simulink model "adas"  (R2022a)
settings: Solver=ode3  StartTime=0.0  StopTime=100  FixedStep=0.02  RelTol=1e-3  EnableMultiTasking=on
undefined symbols (not defined in the file): kd, kp
libraries: simulink x1
settings Model: ExtModeTrigDuration=2  Creator=hp  LastModifiedBy=hp
settings DataIOCC: TimeSaveName=HIL  OutputSaveName=HIL  SignalLoggingName=HILout  DSMLoggingName=HILout
settings OptimizationCC: EnhancedBackFolding=on  PassReuseOutputArgsAs=Individual arguments  ZeroExternalMemoryAtStartup=off  ZeroInternalMemoryAtStartup=off  MaxStackSize=64  OptimizeBlockOrder=speed  DifferentSizesBufferReuse=on  OptimizationCustomize=off  EfficientTunableParamExpr=on
settings DebuggingCC: ParameterTunabilityLossMsg=error
settings HardwareCC: ProdBitPerInt=16  ProdBitPerPointer=16  ProdBitPerSizeT=16  ProdBitPerPtrDiffT=16  ProdLargestAtomicFloat=None  ProdWordSize=8  ProdHWDeviceType=Atmel->AVR
settings SFSimCC: MATLABDynamicMemAlloc=off
settings RTWCC: SystemTargetFile=ert.tlc  HardwareBoard=Arduino Uno  TemplateMakefile=ert_default_tmf  Toolchain=Arduino AVR  BuildConfiguration=Faster Runs  PortableWordSizes=on
settings CodeAppCC: ForceParamTrailComments=on  IgnoreCustomStorageClasses=off  OperatorAnnotations=on  SimulinkDataObjDesc=on  SFDataObjDesc=on  InsertBlockDesc=on
settings ERTTargetCC: SupportContinuousTime=on  SupportVariableSizeSignals=on  ExtModeTransport=3  ExtModeStaticAlloc=on  ExtModeStaticAllocSize=250  ExtModeMexFile=ext_xcp  ExtModeIntrfLevel=Level2 - Open

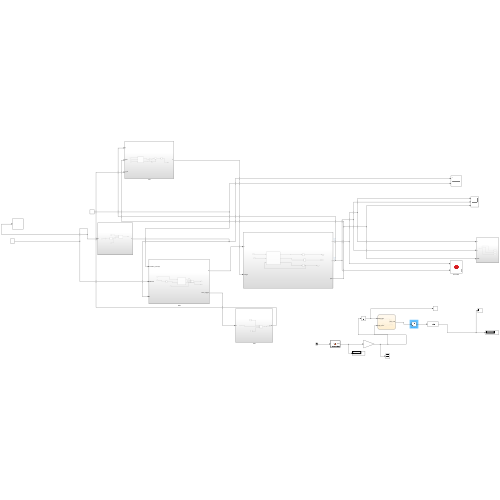
[thumbnail: Simulink's stored preview of the top-level diagram]
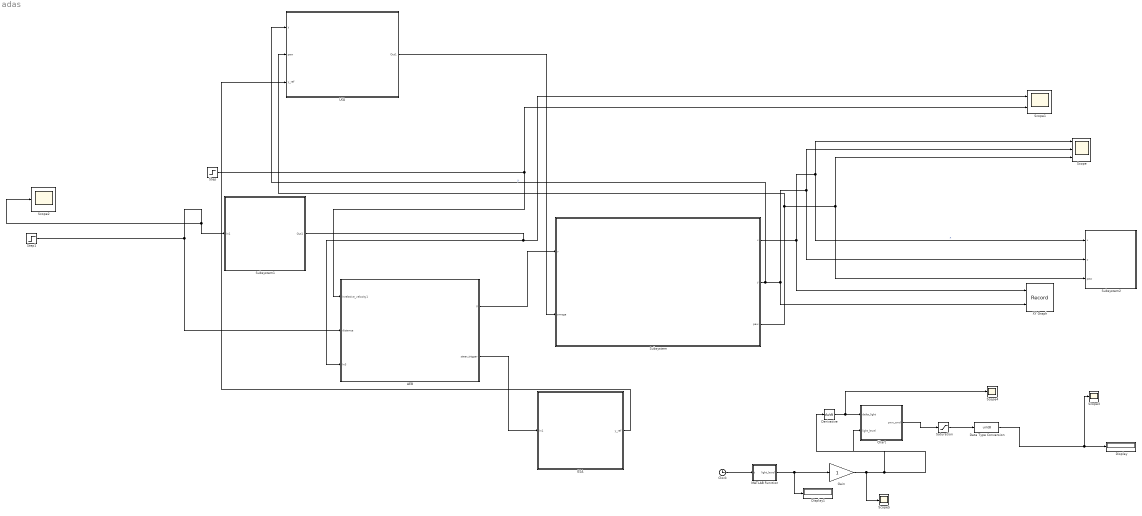
== system adas ==
  AEB : Subsystem
  Chart : Stateflow chart  TreatAsAtomicUnit=on
  Clock : Clock
  Data Type Conversion : DataTypeConversion  OutDataTypeStr=uint8  SaturateOnIntegerOverflow=off  RndMeth=Floor
  Derivative : Derivative
  Display : Display
  Display1 : Display
  ESA : Subsystem
  Gain : Gain  ParamDataTypeStr=double
  LKA : Subsystem
  MATLAB Function : MATLAB Function  TreatAsAtomicUnit=on
  Saturation : Saturate  UpperLimit=255  LowerLimit=0
  Scope : Scope  NumInputPorts=3
  Scope1 : Scope  NumInputPorts=2
  Scope{2..5} (4 alike) : Scope
  Step : Step  Time=5  SampleTime=0.02
  Step1 : Step  Time=45  Before=100  After=5  SampleTime=0.02
  Subsystem : Subsystem
  Subsystem1 : Subsystem
  Subsystem2 : Subsystem
  XY Graph : Record  FileSettingsInternal="{\"entries\":[{\"content\":{\"excelSettings\":{\"content\":{},\"type\":\"Streamout.ExcelSettings\"}},\"type\":\"Streamout.FileSettingStorage\",\"uuid\":\"61d12974-7c49-4c6c-a54c-f09717fa1486\"}],\"packageUris\":[\"http://schema.mathworks.com/mf0/streamout_blocks/R2020a\"],\"version\":\"1.0\"}"  Layout=[1 1]  SignalsInternal="{\"entries\":[{\"content\":{\"signals\":[{\"content\":{\"blockPath\":[\"adas/XY Graph\"],\"channel\":[],\"dimensions\":[1],\"domain\":\"adas/XY Graph\",\"lineColor\":\"#64d413\",\"plots\":[1],\"port\":1,\"sid\":[\"\"],\"signalID\":220,\"signalName\":\"x\"},\"type\":\"RecordBlkView.Signal\",\"uuid\":\"ebedb142-5f9a-4bb0-8b24-e7615f5b49e4\"},{\"content\":{\"blockPath\":[\"adas/XY Graph\"],\"channel\":[],\"dimensions\":[1],\"domain\":\"adas/XY Graph\",\"lineColor\":\"#ff13a6\",\"plots\":[1],\"port\":2,\"sid\":[\"\"],\"signalID\":224,\"signalName\":\"y\"},\"type\":\"RecordBlkView.Signal\",\"uuid\":\"06ee9b17-8867-4135-9d05-b61322aa9b8c\"}]},\"type\":\"RecordBlkView.InputSignals\",\"uuid\":\"24a18c73-a9db-4983-85ff-7d99e9321247\"}],\"packageUris\":[\"http://schema.mathworks.com/mf0/streamout_blocks/R2020a\"],\"version\":\"1.0\"}"  VisualizationBindings="{\"xyplotplugin\":{\"info\":[{\"series\":[{\"bindingParametersList\":[{\"parameter\":\"X-Axis\",\"signalID\":220,\"signalName\":\"x\"},{\"parameter\":\"Y-Axis\",\"signalID\":224,\"signalName\":\"y\"}],\"seriesID\":5354}],\"subplotID\":1}]}}"  CompatibilityTag=XY
  wires:
  Subsystem1/1(Out1) -> AEB/3(In3), Scope1/1
  Subsystem/1(x) -> Subsystem2/1(x), Scope/1, XY Graph/1  "x"
  Subsystem/2(y) -> LKA/1(y), Subsystem2/2(y), Scope/2, XY Graph/2  "y"
  Subsystem/3(paw) -> LKA/2(paw), Subsystem2/3(paw), Scope/3
  Step/1 -> AEB/1(Inrelative_velocity1), Scope1/2
  LKA/1(Out1) -> Subsystem/2(omega)
  Step1/1 -> Scope2/1, Subsystem1/1(In1), AEB/2(distance)
  AEB/1(V) -> Subsystem/1(v)
  AEB/2(steer_trigger) -> ESA/1(In1)
  ESA/1(y_ref) -> LKA/3(y_ref)
  Clock/1 -> MATLAB Function/1(t)
  Derivative/1 -> Scope4/1, Chart/1(delta_light)
  Chart/1(pwn_cmd) -> Saturation/1
  Saturation/1 -> Data Type Conversion/1
  Gain/1 -> Scope5/1, Chart/2(light_level), Derivative/1
  Data Type Conversion/1 -> Scope3/1, Display/1
  MATLAB Function/1(light_level) -> Display1/1, Gain/1

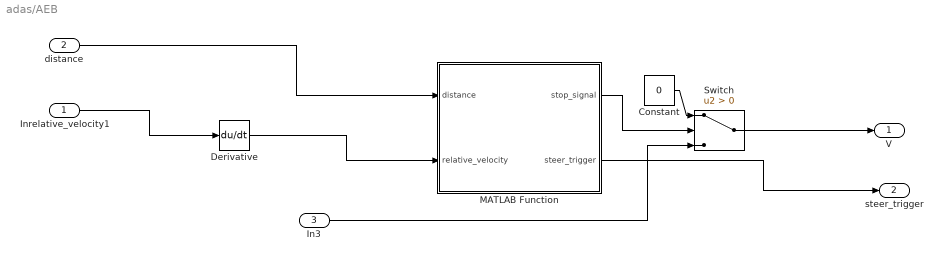
== system adas/AEB ==
  Inrelative_velocity1 : Inport
  distance : Inport  Port=2
  In3 : Inport  Port=3
  Constant : Constant  Value=0  SampleTime=0.02
  Derivative : Derivative
  MATLAB Function : MATLAB Function  TreatAsAtomicUnit=on
  Switch : Switch  Criteria=u2 > Threshold  SaturateOnIntegerOverflow=off  InputSameDT=off
  V : Outport
  steer_trigger : Outport  Port=2
  wires:
  Derivative/1 -> MATLAB Function/2(relative_velocity)
  Constant/1 -> Switch/1
  MATLAB Function/1(stop_signal) -> Switch/2
  distance/1 -> MATLAB Function/1(distance)
  Switch/1 -> V/1
  In3/1 -> Switch/3
  Inrelative_velocity1/1 -> Derivative/1
  MATLAB Function/2(steer_trigger) -> steer_trigger/1

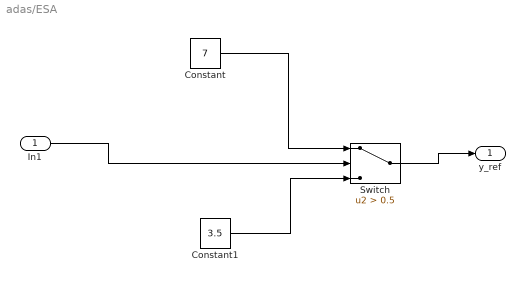
== system adas/ESA ==
  In1 : Inport
  Constant : Constant  Value=7  SampleTime=0.02
  Constant1 : Constant  Value=3.5  SampleTime=0.02
  Switch : Switch  Criteria=u2 > Threshold  Threshold=0.5  SaturateOnIntegerOverflow=off  InputSameDT=off
  y_ref : Outport
  wires:
  Constant1/1 -> Switch/3
  Switch/1 -> y_ref/1
  Constant/1 -> Switch/1
  In1/1 -> Switch/2

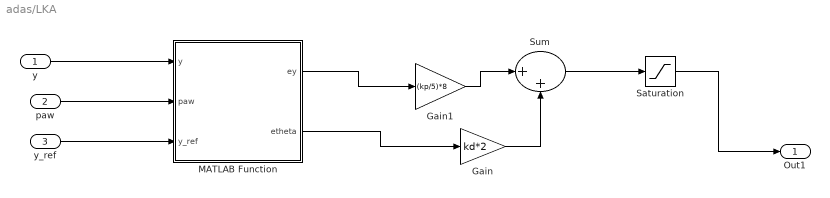
== system adas/LKA ==
  y : Inport
  paw : Inport  Port=2
  y_ref : Inport  Port=3
  Gain : Gain  Gain=kd*2
  Gain1 : Gain  Gain=(kp/5)*8
  MATLAB Function : MATLAB Function  TreatAsAtomicUnit=on
  Saturation : Saturate
  Sum : Sum  Inputs=|++
  Out1 : Outport
  wires:
  paw/1 -> MATLAB Function/2(paw)
  y/1 -> MATLAB Function/1(y)
  Gain/1 -> Sum/2
  Gain1/1 -> Sum/1
  Sum/1 -> Saturation/1
  Saturation/1 -> Out1/1
  MATLAB Function/1(ey) -> Gain1/1
  MATLAB Function/2(etheta) -> Gain/1
  y_ref/1 -> MATLAB Function/3(y_ref)

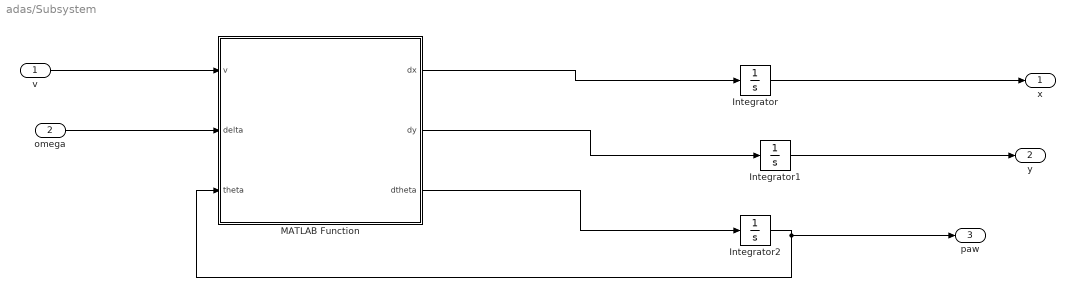
== system adas/Subsystem ==
  v : Inport
  omega : Inport  Port=2
  Integrator : Integrator
  Integrator1 : Integrator
  Integrator2 : Integrator
  MATLAB Function : MATLAB Function  TreatAsAtomicUnit=on
  x : Outport
  y : Outport  Port=2
  paw : Outport  Port=3
  wires:
  Integrator2/1 -> MATLAB Function/3(theta), paw/1
  MATLAB Function/1(dx) -> Integrator/1
  MATLAB Function/2(dy) -> Integrator1/1
  MATLAB Function/3(dtheta) -> Integrator2/1
  v/1 -> MATLAB Function/1(v)
  omega/1 -> MATLAB Function/2(delta)
  Integrator/1 -> x/1
  Integrator1/1 -> y/1

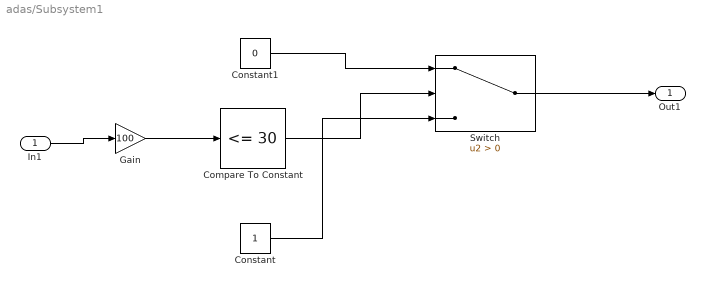
== system adas/Subsystem1 ==
  In1 : Inport
  Compare To Constant : simulink/Logic and Bit Operations/Compare To Constant  relop=<=  const=30  OutDataTypeStr=boolean
  Constant : Constant  SampleTime=0.02
  Constant1 : Constant  Value=0  SampleTime=0.02
  Gain : Gain  Gain=100
  Switch : Switch  Criteria=u2 > Threshold  SaturateOnIntegerOverflow=off  InputSameDT=off
  Out1 : Outport
  wires:
  Constant/1 -> Switch/3
  Compare To Constant/1 -> Switch/2
  Constant1/1 -> Switch/1
  Switch/1 -> Out1/1
  Gain/1 -> Compare To Constant/1
  In1/1 -> Gain/1

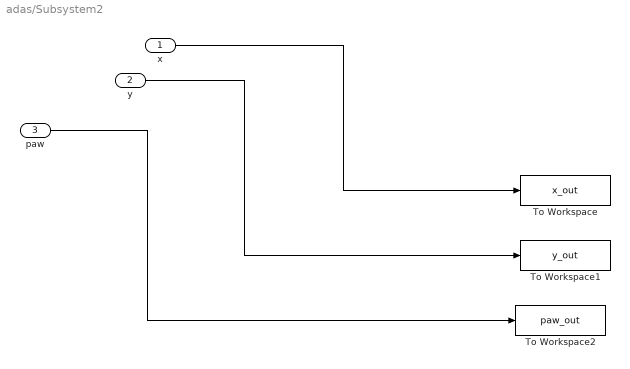
== system adas/Subsystem2 ==
  x : Inport
  y : Inport  Port=2
  paw : Inport  Port=3
  To Workspace : ToWorkspace  VariableName=x_out  SaveFormat=Structure With Time  SampleTime=-1
  To Workspace1 : ToWorkspace  VariableName=y_out  SaveFormat=Structure With Time  SampleTime=-1
  To Workspace2 : ToWorkspace  VariableName=paw_out  SaveFormat=Structure With Time  SampleTime=-1
  wires:
  paw/1 -> To Workspace2/1
  y/1 -> To Workspace1/1
  x/1 -> To Workspace/1

== matlab function adas/LKA/MATLAB Function ==
  data: y input; ey output; paw input; y_ref input; etheta output
function [ey, etheta] = errors(y, paw, y_ref)
    ey = y_ref - y; % Distance perpendiculaire à la voie
    etheta = 0 - paw; % Différence entre l'angle voulu (0 rad) et l'angle actuel
end

== matlab function adas/Subsystem/MATLAB Function ==
  data: v input; dx output; delta input; theta input; dy output; dtheta output
function [dx, dy, dtheta] = robot_bicycle(v, delta, theta)
    
    L = 2.5; 

    dx = v * cos(theta);
    dy = v * sin(theta);

   
    dtheta = (v / L) * tan(delta); 
end

== matlab function adas/AEB/MATLAB Function ==
  data: distance input; stop_signal output; relative_velocity input; steer_trigger output
function [stop_signal, steer_trigger] = TTC_Logic(distance, relative_velocity)
    % On utilise la distance brute pour valider les connexions
    if distance < 15
        steer_trigger = 1; % On commence à tourner si d < 15
    else
        steer_trigger = 0;
    end
    
    if distance < 5
        stop_signal = 1; % On freine si d < 5
    else
        stop_signal = 0;
    end
end

== stateflow chart adas/Chart ==
  state DAY
    en:pwn_cmd=0;
  state DUSK
    en:pwn_cmd=120;
  state TUNNEL
    pwn_cmd=255;
  state NIGHT
    pwn_cmd=220;
  (default) -> DAY
  DAY -> DUSK : [light_level<0.65]
  DUSK -> DAY [order 1] : [light_level>0.75]
  NIGHT -> DUSK [order 1] : [light_level>0.45]
  DUSK -> NIGHT [order 2] : [light_level<0.35]
  TUNNEL -> NIGHT : [after(2,sec) && light_level > 0.4]
  NIGHT -> TUNNEL [order 2] : [delta_light < -0.2]
  data: pwn_cmd output; delta_light input; light_level input

== matlab function adas/MATLAB Function ==
  data: t input; light_level output
function light_level = environment_sim(t)
    if t < 44
        light_level = 1.0;   % JOUR 
    elseif t < 45
        light_level = 0.6;   % DUSK 
    elseif t < 70
        light_level = 0.05;  % TUNNEL 
    else
        light_level = 1.0;   % SORTIE 
    end
end
